simulink model "IonSatSimulation_ne_marche_pas_version_robin-lx-tavant.lab-lpp.local"  (R2019a)
settings: Solver=ode3  StartTime=0.0  StopTime=10000  FixedStep=.25  MaxStep=30  MinStep=.1  RelTol=1e-3
PreLoadFcn:
  | load('.\Data\SatConstants.mat')
model workspace (MAT data in the model file):
  MCOS : class17 (value not decoded)
  MCOS : class17 (value not decoded)
undefined symbols (not defined in the file): Angle, Axis, deg, DiscIntNeverNeededParam, IAU, km, m, mu_Earth, rad, s, sat, X, Y, Z
libraries: aerolibutil x29, sm_lib x19, nesl_utility x16, aerolibconvert2 x13, vrlib x10, simulink x9, dspmathops x8, sharedtransform x7, sharedutil x5, aerolibgravity2 x4, sharedTrackingLibrary x2, aerolibcelestial x2
(part 3 of 3)

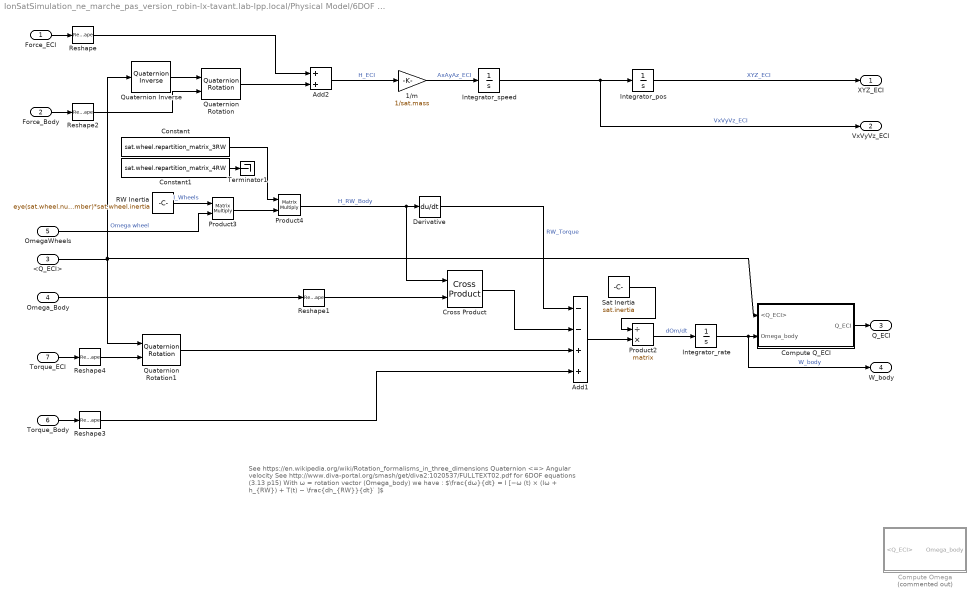
== system IonSatSimulation_ne_marche_pas_version_robin-lx-tavant.lab-lpp.local/Physical Model/6DOF in ECI frame ==
  note: See https://en.wikipedia.org/wiki/Rotation_formalisms_in_three_dimensions Quaternion <=> Angular velocity
      |
      | See http://www.diva-portal.org/smash/get/diva2:1020537/FULLTEXT02.pdf for 6DOF equations (3.13 p15)
      |
      | With ω = rotation vector (Omega_body) we have :
      |
      | $\frac{dω}{dt} = I [−ω (t) × (Iω + h_{RW}) + T(t) − \frac{dh_{RW}}{dt} ̇ ]$
  Force_ECI : Inport
  Force_Body : Inport  Port=2
  <Q_ECI> : Inport  Port=3
  "Omega_Body " : Inport  Port=4
  OmegaWheels : Inport  Port=5
  Torque_Body : Inport  Port=6
  Torque_ECI : Inport  Port=7  PortDimensions=3
  1/m : Gain  Gain=1/sat.mass
  Add1 : Sum  Inputs=--++
  Add2 : Sum
  Compute Omega : Subsystem  Commented=on
  Compute Q_ECI : Subsystem
  Constant : Constant  Value=sat.wheel.repartition_matrix_3RW
  Constant1 : Constant  Value=sat.wheel.repartition_matrix_4RW
  Cross Product : vrlib/Utilities/Cross Product
      settings: SourceProductName=Simulink
  Derivative : Derivative
  Integrator_pos : Integrator
  Integrator_rate : Integrator
  Integrator_speed : Integrator
  Product2 : Product  Inputs=/*  Multiplication=Matrix(*)
  Product3 : Product  Multiplication=Matrix(*)
  Product4 : Product  Multiplication=Matrix(*)
  Quaternion Inverse : aerolibutil/Quaternion Inverse
      settings: SourceProductName=Aerospace Blockset
  Quaternion Rotation : aerolibutil/Quaternion Rotation
  Quaternion Rotation1 : aerolibutil/Quaternion Rotation
  RW Inertia : Constant  Value=eye(sat.wheel.number)*sat.wheel.inertia
  Reshape{,1..4} (5 alike) : Reshape  OutputDimensionality=Column vector (2-D)
  Sat Inertia : Constant  Value=sat.inertia
  Terminator1 : Terminator
  XYZ_ECI : Outport
  VxVyVz_ECI : Outport  Port=2
  Q_ECI : Outport  Port=3
  W_body : Outport  Port=4
  wires:
  Product2/1 -> Integrator_rate/1  "dOm/dt"
  Product3/1 -> Product4/2
  Sat Inertia/1 -> Product2/1
  Add1/1 -> Product2/2
  Cross Product/1 -> Add1/2
  "Omega_Body "/1 -> Reshape1/1
  Integrator_rate/1 -> W_body/1, Compute Q_ECI/2(Omega_body)  "W_body"
  RW Inertia/1 -> Product3/1  "I_Wheels"
  Torque_Body/1 -> Reshape3/1
  Derivative/1 -> Add1/1  "RW_Torque"
  OmegaWheels/1 -> Product3/2  "Omega wheel"
  Compute Q_ECI/1(Q_ECI) -> Q_ECI/1
  1/m/1 -> Integrator_speed/1  "AxAyAz_ECI"
  Integrator_pos/1 -> XYZ_ECI/1  "XYZ_ECI"
  Integrator_speed/1 -> VxVyVz_ECI/1, Integrator_pos/1  "VxVyVz_ECI"
  Force_Body/1 -> Reshape2/1
  Quaternion Inverse/1 -> Quaternion Rotation/1
  Add2/1 -> 1/m/1  "H_ECI"
  Quaternion Rotation/1 -> Add2/2
  Force_ECI/1 -> Reshape/1
  Torque_ECI/1 -> Reshape4/1
  <Q_ECI>/1 -> Quaternion Rotation1/1, Quaternion Inverse/1, Compute Q_ECI/1(<Q_ECI>)
  Quaternion Rotation1/1 -> Add1/3
  Constant1/1 -> Terminator1/1
  Constant/1 -> Product4/1
  Reshape/1 -> Add2/1
  Reshape2/1 -> Quaternion Rotation/2
  Reshape3/1 -> Add1/4
  Reshape4/1 -> Quaternion Rotation1/2
  Product4/1 -> Cross Product/1, Derivative/1  "H_RW_Body"
  Reshape1/1 -> Cross Product/2

== system IonSatSimulation_ne_marche_pas_version_robin-lx-tavant.lab-lpp.local/Physical Model/Magnetorquer physics ==
  note: On pourrait aussi changer les blocs
      | magnétocoupleurs pour sortir les intensités
  Mag vector command : Inport
  B_IGRF_body (vecteur) : Inport  Port=2
  Add1 : Sum  Inputs=+++
  Cross Product : vrlib/Utilities/Cross Product
      settings: SourceProductName=Simulink
  Demux : Demux  Outputs=3
  Magnétocoupleur 1 : Subsystem
  Magnétocoupleur 2 : Subsystem
  Magnétocoupleur 3 : Subsystem
  Couple (vect) : Outport  PortDimensions=3
  Real mag moments vector : Outport  Port=2
  wires:
  Add1/1 -> Real mag moments vector/1, Cross Product/1  "M_real"
  Demux/1 -> Magnétocoupleur 1/1(m_in (scalar))
  Demux/2 -> Magnétocoupleur 2/1(m_in (scalar))
  Demux/3 -> Magnétocoupleur 3/1(m_in (scalar))
  Mag vector command/1 -> Demux/1
  Magnétocoupleur 2/1(m_out (vect)) -> Add1/2
  Magnétocoupleur 1/1(m_out (vect)) -> Add1/1
  Magnétocoupleur 3/1(m_out (vect)) -> Add1/3
  Cross Product/1 -> Couple (vect)/1  "T_body"
  B_IGRF_body (vecteur)/1 -> Cross Product/2

== system IonSatSimulation_ne_marche_pas_version_robin-lx-tavant.lab-lpp.local/Physical Model/RW physics ==
  RW command : Inport
  Demux : Demux  Outputs=3
  Mux : Mux  Inputs=3
  Transfer Fcn : TransferFcn  Denominator=[1 1]
  Transfer Fcn1 : TransferFcn  Denominator=[1 1]
  Transfer Fcn2 : TransferFcn  Denominator=[1 1]
  RW speed : Outport
  wires:
  Demux/3 -> Transfer Fcn2/1
  Demux/2 -> Transfer Fcn1/1
  Transfer Fcn2/1 -> Mux/3
  Transfer Fcn1/1 -> Mux/2
  Demux/1 -> Transfer Fcn/1
  Transfer Fcn/1 -> Mux/1
  RW command/1 -> Demux/1
  Mux/1 -> RW speed/1

== system IonSatSimulation_ne_marche_pas_version_robin-lx-tavant.lab-lpp.local/Physical Model/Spherical Harmonic Gravity ==
  note: Slower subsytem because it's too slow
  XYZ_ECI : Inport
  Time_UTC : Inport  Port=2
  ECI to ECEF IAU-2000/2006 : MATLAB Function  TreatAsAtomicUnit=on
  Product : Product  Multiplication=Matrix(*)
  Product1 : Product  Inputs=/*  Multiplication=Matrix(*)
  Spherical Harmonic Gravity Model : aerolibgravity2/Spherical Harmonic Gravity Model  units=Metric (MKS)  degree=100  action=Warning  ptype=EGM2008  datafile='aerogmm2b.mat'
      settings: SourceProductName=Aerospace Blockset  SourceProductBaseCode=AE
  Transpose : Math  Operator=transpose  SaturateOnIntegerOverflow=on
  g_ECI (m/s²) : Outport  VectorParamsAs1DForOutWhenUnconnected=on
  wires:
  ECI to ECEF IAU-2000/2006/1(DCM) -> Product1/1, Product/1
  Transpose/1 -> Product1/2
  Product/1 -> Spherical Harmonic Gravity Model/1
  Spherical Harmonic Gravity Model/1 -> Transpose/1
  XYZ_ECI/1 -> Product/2
  Product1/1 -> g_ECI (m/s²)/1
  Time_UTC/1 -> ECI to ECEF IAU-2000/2006/1(Time_UTC)

== system IonSatSimulation_ne_marche_pas_version_robin-lx-tavant.lab-lpp.local/Physical Model/Thruster ==
  On/Off (Boolean) : Inport  OutDataTypeStr=boolean
  Constant : Constant  Value=0
  Cross Product : vrlib/Utilities/Cross Product
      settings: SourceProductName=Simulink
  If : If  IfExpression=u1
  If Action Subsystem : Subsystem  TreatAsAtomicUnit=on
  If Action Subsystem1 : Subsystem  TreatAsAtomicUnit=on
  Merge : Merge
  Product : Product
  Thruster Force : Constant  Value=sat.thruster.force
  unit vector of thrust : Constant  Value=sat.thruster.dir
  vector G-Thrust point : Constant  Value=sat.thruster.point
  Force (G_sat) : Outport
  Moment (G_sat) : Outport  Port=2
  wires:
  Product/1 -> Force (G_sat)/1, Cross Product/2
  vector G-Thrust point/1 -> Cross Product/1
  unit vector of thrust/1 -> Product/1
  Cross Product/1 -> Moment (G_sat)/1
  Thruster Force/1 -> If Action Subsystem/1(In1)
  On/Off (Boolean)/1 -> If/1
  If/1 -> If Action Subsystem/Action
  If/2 -> If Action Subsystem1/Action
  If Action Subsystem1/1(Out1) -> Merge/2
  If Action Subsystem/1(Out1) -> Merge/1
  Merge/1 -> Product/2
  Constant/1 -> If Action Subsystem1/1(In1)

== system IonSatSimulation_ne_marche_pas_version_robin-lx-tavant.lab-lpp.local/Sensors/MEMS Gyro ==
  note: Voir ICD sur le CubeControl (pas 100% sur néanmoins)
  U : Inport
  Bus Selector4 : BusSelector  OutputSignals=W_body
  Constant : Constant  Value=[sat.sensors.gyro_bias sat.sensors.gyro_bias sat.sensors.gyro_bias]
  Random Number : RandomNumber  Mean=[0 0 0]  Variance=sat.sensors.mag_sigma*sat.sensors.mag_sigma  Seed=[0 5 355]  SampleTime=1
  Reshape : Reshape  OutputDimensionality=Column vector (2-D)
  Reshape1 : Reshape  OutputDimensionality=Column vector (2-D)
  Sum : Sum  Inputs=|++
  Sum1 : Sum  Inputs=|++
  W_Body_meas : Outport
  wires:
  U/1 -> Bus Selector4/1
  Random Number/1 -> Reshape/1
  Sum/1 -> Sum1/1
  Reshape/1 -> Sum/2  "Noise"
  Bus Selector4/1 -> Sum/1  "<W_body>"
  Sum1/1 -> W_Body_meas/1
  Constant/1 -> Reshape1/1
  Reshape1/1 -> Sum1/2  "Bias"

== system IonSatSimulation_ne_marche_pas_version_robin-lx-tavant.lab-lpp.local/Sensors/Magnetometer ==
  note: Valeur constructeur : 1-sigma = 50nT
  U : Inport
  B_IGRF_ECI : Inport  Port=2
  Bus Selector : BusSelector  OutputSignals=Q_ECI
  Quaternion Rotation : aerolibutil/Quaternion Rotation
  Random Number : RandomNumber  Mean=[0 0 0]  Variance=sat.sensors.mag_sigma*sat.sensors.mag_sigma  Seed=[0 5 355]  SampleTime=1
  Reshape : Reshape  OutputDimensionality=Column vector (2-D)
  Sum : Sum  Inputs=|++
  B_Body_meas : Outport
  wires:
  B_IGRF_ECI/1 -> Quaternion Rotation/2
  Random Number/1 -> Reshape/1
  Quaternion Rotation/1 -> Sum/1  "B_IGRF_body"
  Sum/1 -> B_Body_meas/1
  Reshape/1 -> Sum/2
  U/1 -> Bus Selector/1
  Bus Selector/1 -> Quaternion Rotation/1  "<Q_ECI>"

== system IonSatSimulation_ne_marche_pas_version_robin-lx-tavant.lab-lpp.local/Sensors/Sun Sensor (Coarse) ==
  note: Tests if we are not in eclipse
  note: Test d'eclipse (true = soleil visible)
  note: Two sensors because the top-camera has a 3-sigma=0.2° wheread the coarse sun sensors have sigma = 10°
  Sat-Sun_ECI : Inport
  U : Inport  Port=2
  Bus Selector : BusSelector  OutputSignals=Q_ECI,XYZ_ECI
  Constant : Constant  Value=true
  Constant1 : Constant  Value=false
  Dot Product : DotProduct  InputSameDT=on  OutDataTypeStr=Inherit: Inherit via internal rule
  Quaternion Rotation : aerolibutil/Quaternion Rotation
  Quaternion Rotation1 : aerolibutil/Quaternion Rotation
  Random Number : RandomNumber  Mean=[0 0 0]  Variance=sat.sensors.sun_coarse_sigma*sat.sensors.sun_coarse_sigma  Seed=[0 5 355]  SampleTime=1  VectorParams1D=off
  Rotation Angles to Quaternions : sharedtransform/Rotation Angles to Quaternions  rotationOrder=ZYX  aMode=aMode
      settings: SourceProductName=Aerospace Blockset  SourceProductBaseCode=AE
  Switch1 : Switch  Criteria=u2 > Threshold
  Sat-Sun_coarse_body_meas : Outport
  Sensor active (bool) : Outport  Port=2
  wires:
  Rotation Angles to Quaternions/1 -> Quaternion Rotation/1
  Quaternion Rotation/1 -> Sat-Sun_coarse_body_meas/1
  U/1 -> Bus Selector/1
  Sat-Sun_ECI/1 -> Dot Product/1, Quaternion Rotation1/2
  Bus Selector/1 -> Quaternion Rotation1/1  "<Q_ECI>"
  Quaternion Rotation1/1 -> Quaternion Rotation/2  "Sat_Sun_body"
  Bus Selector/2 -> Dot Product/2  "<XYZ_ECI>"
  Dot Product/1 -> Switch1/2
  Constant/1 -> Switch1/1
  Constant1/1 -> Switch1/3
  Switch1/1 -> Sensor active (bool)/1
  Random Number/1 -> Rotation Angles to Quaternions/1

== system IonSatSimulation_ne_marche_pas_version_robin-lx-tavant.lab-lpp.local/Sensors/Sun Sensor (Sun sensor) ==
  note: Tests if the camera is seeing the sun
  note: Test d'eclipse
  note: Two sensors because the top-camera has a 3-sigma=0.2° wheread the coarse sun sensors have sigma = 10°
  note: Valeur constructeur : 3-sigma = 0.2°
      | Donc sigma = 0.066° = 0.001164 rad
  Sat-Sun_ECI : Inport
  U : Inport  Port=2
  AND : Logic  IconShape=distinctive  AllPortsSameDT=off  OutDataTypeStr=boolean
  Bus Selector : BusSelector  OutputSignals=Q_ECI,XYZ_ECI
  Constant : Constant  Value=true
  Constant1 : Constant  Value=false
  Constant3 : Constant  Value=true
  Constant4 : Constant  Value=false
  Demux : Demux  Outputs=3
  Dot Product : DotProduct  InputSameDT=on  OutDataTypeStr=Inherit: Inherit via internal rule
  Quaternion Rotation : aerolibutil/Quaternion Rotation
  Quaternion Rotation1 : aerolibutil/Quaternion Rotation
  Random Number : RandomNumber  Mean=[0 0 0]  Variance=sat.sensors.sun_sigma*sat.sensors.sun_sigma  Seed=[0 5 355]  SampleTime=1  VectorParams1D=off
  Rotation Angles to Quaternions : sharedtransform/Rotation Angles to Quaternions  rotationOrder=ZYX  aMode=aMode
      settings: SourceProductName=Aerospace Blockset  SourceProductBaseCode=AE
  Switch : Switch  Criteria=u2 > Threshold
  Switch1 : Switch  Criteria=u2 > Threshold
  Terminator : Terminator
  Terminator1 : Terminator
  Sat-Sun_precise_body_meas : Outport
  Sensor active (bool) : Outport  Port=2
  wires:
  Switch/1 -> AND/1
  Rotation Angles to Quaternions/1 -> Quaternion Rotation/1
  Quaternion Rotation/1 -> Sat-Sun_precise_body_meas/1
  U/1 -> Bus Selector/1
  Sat-Sun_ECI/1 -> Dot Product/1, Quaternion Rotation1/2
  Bus Selector/1 -> Quaternion Rotation1/1  "<Q_ECI>"
  Quaternion Rotation1/1 -> Demux/1, Quaternion Rotation/2  "Sat_Sun_body"
  Demux/3 -> Switch/2
  Constant3/1 -> Switch/1
  Demux/2 -> Terminator/1
  Demux/1 -> Terminator1/1
  Bus Selector/2 -> Dot Product/2  "<XYZ_ECI>"
  Dot Product/1 -> Switch1/2
  Constant/1 -> Switch1/1
  Constant1/1 -> Switch1/3
  Switch1/1 -> AND/2
  AND/1 -> Sensor active (bool)/1
  Random Number/1 -> Rotation Angles to Quaternions/1
  Constant4/1 -> Switch/3

== system IonSatSimulation_ne_marche_pas_version_robin-lx-tavant.lab-lpp.local/Controller/B-dot choice1/Switch Case Action Subsystem3 ==
  In1 : Inport
  Action Port : ActionPort  ActionPortLabel=if(u1 > 0)
  Out1 : Outport
  wires:
  In1/1 -> Out1/1

== system IonSatSimulation_ne_marche_pas_version_robin-lx-tavant.lab-lpp.local/Controller/B-dot choice1/Switch Case Action Subsystem4 ==
  In1 : Inport
  Action Port : ActionPort  ActionPortLabel=else
  Out1 : Outport
  wires:
  In1/1 -> Out1/1

== system IonSatSimulation_ne_marche_pas_version_robin-lx-tavant.lab-lpp.local/Controller/B-dot choice2/Switch Case Action Subsystem3 ==
  In1 : Inport
  Action Port : ActionPort  ActionPortLabel=if(u1 > 0)
  Out1 : Outport
  wires:
  In1/1 -> Out1/1

== system IonSatSimulation_ne_marche_pas_version_robin-lx-tavant.lab-lpp.local/Controller/B-dot choice2/Switch Case Action Subsystem4 ==
  In1 : Inport
  Action Port : ActionPort  ActionPortLabel=else
  Out1 : Outport
  wires:
  In1/1 -> Out1/1

== system IonSatSimulation_ne_marche_pas_version_robin-lx-tavant.lab-lpp.local/Controller/PID (nominal command)/Command Magnetic moments computation ==
  note: Moment magnétique de commande M :
      |
      | $M_c = \frac{1}{B²}\vec{B} \wedge\vec{T_P}$
      |
      | Avec Tp couple projeté dans le plan orthogonal à B
      | $T_P=\vec{T}-\frac{1}{B²}(\vec{T}\cdot\vec{B})\vec{B}$
  Command (vect) : Inport  OutDataTypeStr=double
  B_IGRF_body (vect) : Inport  Port=2  OutDataTypeStr=double
  h1 (vect) : Inport  Port=3
  h2 (vect) : Inport  Port=4
  h3 (vect) : Inport  Port=5
  Cross Product : vrlib/Utilities/Cross Product
      settings: SourceProductName=Simulink
  Dot Product : DotProduct  InputSameDT=on  OutDataTypeStr=Inherit: Inherit via internal rule
  Global magnetic moment computation : Subsystem
  Mux : Mux  Inputs=3
  Product1 : Product  Inputs=*/
  Reshape : Reshape  OutputDimensionality=Column vector (2-D)
  Reshape1 : Reshape  OutputDimensionality=Column vector (2-D)
  Mag vector command : Outport
  wires:
  B_IGRF_body (vect)/1 -> Reshape1/1  "B_Body"
  Command (vect)/1 -> Reshape/1  "T_Body"
  h1 (vect)/1 -> Global magnetic moment computation/2(In2)
  h2 (vect)/1 -> Global magnetic moment computation/3(In3)
  h3 (vect)/1 -> Global magnetic moment computation/4(In4)
  Global magnetic moment computation/2(magnetic moment 2 (scalar)) -> Mux/2  "magnetic moment 2"
  Global magnetic moment computation/3(magnetic moment 3 (scalar)) -> Mux/3  "magnetic moment 3"
  Global magnetic moment computation/1(magnetic moment 1 (scalar)) -> Mux/1  "magnetic moment 1"
  Mux/1 -> Mag vector command/1
  Reshape1/1 -> Cross Product/1, Dot Product/2, Dot Product/1
  Cross Product/1 -> Product1/1
  Product1/1 -> Global magnetic moment computation/1(In1)  "Mc"
  Dot Product/1 -> Product1/2  "B^2"
  Reshape/1 -> Cross Product/2  "Tp"

== system IonSatSimulation_ne_marche_pas_version_robin-lx-tavant.lab-lpp.local/Controller/PID (nominal command)/Extract Vect ==
  Qr : Inport
  Demux : Demux
  Mux1 : Mux  Inputs=3
  Product : Product
  Reshape : Reshape  OutputDimensionality=Column vector (2-D)
  Sign : Signum
  Qvect : Outport
  wires:
  Demux/2 -> Mux1/1
  Demux/4 -> Mux1/3
  Demux/3 -> Mux1/2
  Demux/1 -> Sign/1
  Qr/1 -> Demux/1
  Mux1/1 -> Product/2
  Product/1 -> Reshape/1
  Sign/1 -> Product/1
  Reshape/1 -> Qvect/1

== system IonSatSimulation_ne_marche_pas_version_robin-lx-tavant.lab-lpp.local/Controller/PID (nominal command)/RW1 ==
  note: Entrées:
      | - Moment de commande (déjà projeté sur l'axe de la roue...)
      | Sorties:
      | - Omega de commande à appliquer
  Mc (scalar) : Inport
  Discrete-Time Integrator : DiscreteIntegrator  IntegratorMethod=Integration: Trapezoidal  SampleTime=-1  ICPrevOutput=DiscIntNeverNeededParam  ICPrevScaledInput=DiscIntNeverNeededParam
  Divide : Product  Inputs=*/
  Saturation_speed : Saturate  UpperLimit=sat.wheel.max_speed  LowerLimit=- sat.wheel.max_speed
  Torque_sat : Saturate  UpperLimit=sat.wheel.max_torque  LowerLimit=- sat.wheel.max_torque
  Wheel Inertia : Constant  Value=sat.wheel.max_sigma/sat.wheel.max_speed
  Omega_C (scalar) : Outport  VectorParamsAs1DForOutWhenUnconnected=on
  wires:
  Wheel Inertia/1 -> Divide/2
  Divide/1 -> Discrete-Time Integrator/1  "dw/dt"
  Discrete-Time Integrator/1 -> Saturation_speed/1
  Torque_sat/1 -> Divide/1  "Torque (scal)"
  Saturation_speed/1 -> Omega_C (scalar)/1
  Mc (scalar)/1 -> Torque_sat/1

== system IonSatSimulation_ne_marche_pas_version_robin-lx-tavant.lab-lpp.local/Controller/PID (nominal command)/RW2 ==
  note: Entrées:
      | - Moment de commande (déjà projeté sur l'axe de la roue...)
      | Sorties:
      | - Omega de commande à appliquer
  Mc (scalar) : Inport
  Discrete-Time Integrator : DiscreteIntegrator  IntegratorMethod=Integration: Trapezoidal  SampleTime=-1  ICPrevOutput=DiscIntNeverNeededParam  ICPrevScaledInput=DiscIntNeverNeededParam
  Divide : Product  Inputs=*/
  Saturation_speed : Saturate  UpperLimit=sat.wheel.max_speed  LowerLimit=- sat.wheel.max_speed
  Torque_sat : Saturate  UpperLimit=sat.wheel.max_torque  LowerLimit=- sat.wheel.max_torque
  Wheel Inertia : Constant  Value=sat.wheel.max_sigma/sat.wheel.max_speed
  Omega_C (scalar) : Outport  VectorParamsAs1DForOutWhenUnconnected=on
  wires:
  Wheel Inertia/1 -> Divide/2
  Divide/1 -> Discrete-Time Integrator/1  "dw/dt"
  Discrete-Time Integrator/1 -> Saturation_speed/1
  Torque_sat/1 -> Divide/1  "Torque (scal)"
  Saturation_speed/1 -> Omega_C (scalar)/1
  Mc (scalar)/1 -> Torque_sat/1

== system IonSatSimulation_ne_marche_pas_version_robin-lx-tavant.lab-lpp.local/Controller/PID (nominal command)/RW3 ==
  note: Entrées:
      | - Moment de commande (déjà projeté sur l'axe de la roue...)
      | Sorties:
      | - Omega de commande à appliquer
  Mc (scalar) : Inport
  Discrete-Time Integrator : DiscreteIntegrator  IntegratorMethod=Integration: Trapezoidal  SampleTime=-1  ICPrevOutput=DiscIntNeverNeededParam  ICPrevScaledInput=DiscIntNeverNeededParam
  Divide : Product  Inputs=*/
  Saturation_speed : Saturate  UpperLimit=sat.wheel.max_speed  LowerLimit=- sat.wheel.max_speed
  Torque_sat : Saturate  UpperLimit=sat.wheel.max_torque  LowerLimit=- sat.wheel.max_torque
  Wheel Inertia : Constant  Value=sat.wheel.max_sigma/sat.wheel.max_speed
  Omega_C (scalar) : Outport  VectorParamsAs1DForOutWhenUnconnected=on
  wires:
  Wheel Inertia/1 -> Divide/2
  Divide/1 -> Discrete-Time Integrator/1  "dw/dt"
  Discrete-Time Integrator/1 -> Saturation_speed/1
  Torque_sat/1 -> Divide/1  "Torque (scal)"
  Saturation_speed/1 -> Omega_C (scalar)/1
  Mc (scalar)/1 -> Torque_sat/1

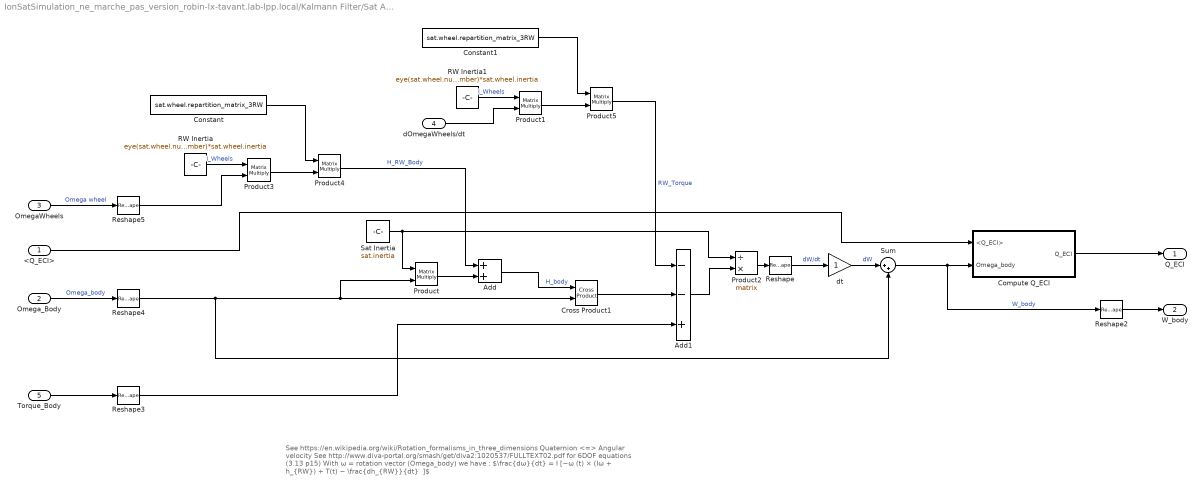
== system IonSatSimulation_ne_marche_pas_version_robin-lx-tavant.lab-lpp.local/Kalmann Filter/Sat Attitude/6DOF in ECI frame ==
  note: See https://en.wikipedia.org/wiki/Rotation_formalisms_in_three_dimensions Quaternion <=> Angular velocity
      |
      | See http://www.diva-portal.org/smash/get/diva2:1020537/FULLTEXT02.pdf for 6DOF equations (3.13 p15)
      |
      | With ω = rotation vector (Omega_body) we have :
      |
      | $\frac{dω}{dt} = I [−ω (t) × (Iω + h_{RW}) + T(t) − \frac{dh_{RW}}{dt} ̇ ]$
  <Q_ECI> : Inport
  "Omega_Body " : Inport  Port=2
  OmegaWheels : Inport  Port=3
  dOmegaWheels/dt : Inport  Port=4
  Torque_Body : Inport  Port=5
  Add : Sum
  Add1 : Sum  Inputs=--+
  Compute Q_ECI : Subsystem
  Constant : Constant  Value=sat.wheel.repartition_matrix_3RW
  Constant1 : Constant  Value=sat.wheel.repartition_matrix_3RW
  Cross Product1 : vrlib/Utilities/Cross Product
      settings: SourceProductName=Simulink
  Product{,1,3..5} (5 alike) : Product  Multiplication=Matrix(*)
  Product2 : Product  Inputs=/*  Multiplication=Matrix(*)
  RW Inertia : Constant  Value=eye(sat.wheel.number)*sat.wheel.inertia
  RW Inertia1 : Constant  Value=eye(sat.wheel.number)*sat.wheel.inertia
  Reshape : Reshape
  Reshape2 : Reshape
  Reshape3 : Reshape  OutputDimensionality=Column vector (2-D)
  Reshape4 : Reshape  OutputDimensionality=Column vector (2-D)
  Reshape5 : Reshape  OutputDimensionality=Column vector (2-D)
  Sat Inertia : Constant  Value=sat.inertia
  Sum : Sum  Inputs=|++
  dt : Gain
  Q_ECI : Outport
  W_body : Outport  Port=2
  wires:
  Product2/1 -> Reshape/1
  Product3/1 -> Product4/2
  Sat Inertia/1 -> Product/1, Product2/1
  Add/1 -> Cross Product1/1  "H_body"
  Add1/1 -> Product2/2
  Cross Product1/1 -> Add1/2
  "Omega_Body "/1 -> Reshape4/1  "Omega_body"
  Product/1 -> Add/2
  RW Inertia/1 -> Product3/1  "I_Wheels"
  Torque_Body/1 -> Reshape3/1
  Product5/1 -> Add1/1  "RW_Torque"
  OmegaWheels/1 -> Reshape5/1  "Omega wheel"
  Constant/1 -> Product4/1
  Product4/1 -> Add/1  "H_RW_Body"
  Reshape3/1 -> Add1/3
  Reshape/1 -> dt/1  "dW/dt"
  Sum/1 -> Compute Q_ECI/2(Omega_body), Reshape2/1  "W_body"
  Compute Q_ECI/1(Q_ECI) -> Q_ECI/1
  Reshape2/1 -> W_body/1
  Reshape4/1 -> Sum/2, Cross Product1/2, Product/2
  Reshape5/1 -> Product3/2
  <Q_ECI>/1 -> Compute Q_ECI/1(<Q_ECI>)
  dt/1 -> Sum/1  "dW"
  dOmegaWheels/dt/1 -> Product1/2
  Constant1/1 -> Product5/1
  Product1/1 -> Product5/2
  RW Inertia1/1 -> Product1/1  "I_Wheels"

== system IonSatSimulation_ne_marche_pas_version_robin-lx-tavant.lab-lpp.local/Kalmann Filter/Sat Attitude/Magnetorquer physics ==
  note: On pourrait aussi changer les blocs
      | magnétocoupleurs pour sortir les intensités
  Mag vector command : Inport
  B_IGRF_body (vecteur) : Inport  Port=2
  Add1 : Sum  Inputs=+++
  Cross Product : vrlib/Utilities/Cross Product
      settings: SourceProductName=Simulink
  Demux : Demux  Outputs=3
  Magnétocoupleur 1 : Subsystem
  Magnétocoupleur 2 : Subsystem
  Magnétocoupleur 3 : Subsystem
  Couple (vect) : Outport
  wires:
  Add1/1 -> Cross Product/1  "M_real"
  Demux/1 -> Magnétocoupleur 1/1(m_in (scalar))
  Demux/2 -> Magnétocoupleur 2/1(m_in (scalar))
  Demux/3 -> Magnétocoupleur 3/1(m_in (scalar))
  Mag vector command/1 -> Demux/1
  Magnétocoupleur 2/1(m_out (vect)) -> Add1/2
  Magnétocoupleur 1/1(m_out (vect)) -> Add1/1
  Magnétocoupleur 3/1(m_out (vect)) -> Add1/3
  Cross Product/1 -> Couple (vect)/1  "T_body"
  B_IGRF_body (vecteur)/1 -> Cross Product/2

== system IonSatSimulation_ne_marche_pas_version_robin-lx-tavant.lab-lpp.local/Kalmann Filter/Sat Attitude1/Compute Q_ECI ==
  note: https://arxiv.org/pdf/0811.2889.pdf
      | $ω = 2q^*\frac{dq}{dt}$ (13)
      |
      | $\frac{dq}{dt} = \frac{1}{2} q * ω$ (14)
  <Q_ECI> : Inport
  Omega_body : Inport  Port=2
  Gain : Gain  Gain=1/2
  Ground : Ground
  Mux : Mux  Inputs=2
  Quaternion Multiplication : aerolibutil/Quaternion Multiplication
  Quaternion Normalize : sharedutil/Quaternion Normalize  aMode=aMode
      settings: SourceProductName=Aerospace Blockset  SourceProductBaseCode=AE
  Sum : Sum  Inputs=|++
  dt : Gain
  Q_ECI : Outport
  wires:
  Quaternion Multiplication/1 -> Gain/1
  Omega_body/1 -> Mux/2
  Ground/1 -> Mux/1
  Mux/1 -> Quaternion Multiplication/2
  Quaternion Normalize/1 -> Q_ECI/1  "Q_ECI"
  Sum/1 -> Quaternion Normalize/1
  <Q_ECI>/1 -> Quaternion Multiplication/1, Sum/1
  Gain/1 -> dt/1  "dQ"
  dt/1 -> Sum/2

== system IonSatSimulation_ne_marche_pas_version_robin-lx-tavant.lab-lpp.local/Physical Model/6DOF in ECI frame/Compute Omega ==
  note: https://arxiv.org/pdf/0811.2889.pdf
      | $ω = 2q^*\frac{dq}{dt}$ (13)
  <Q_ECI> : Inport
  Demux : Demux  Outputs=2
  Derivative : Derivative
  Gain : Gain  Gain=2
  Quaternion Conjugate : aerolibutil/Quaternion Conjugate
      settings: SourceProductName=Aerospace Blockset  SourceProductBaseCode=AE
  Quaternion Multiplication : aerolibutil/Quaternion Multiplication
  Reshape : Reshape  OutputDimensionality=Column vector (2-D)
  Terminator : Terminator
  Omega_body : Outport  PortDimensions=[3 1]
  wires:
  Quaternion Multiplication/1 -> Demux/1
  <Q_ECI>/1 -> Derivative/1, Quaternion Conjugate/1
  Demux/1 -> Terminator/1
  Demux/2 -> Reshape/1
  Reshape/1 -> Gain/1
  Gain/1 -> Omega_body/1
  Quaternion Conjugate/1 -> Quaternion Multiplication/1
  Derivative/1 -> Quaternion Multiplication/2

== system IonSatSimulation_ne_marche_pas_version_robin-lx-tavant.lab-lpp.local/Physical Model/6DOF in ECI frame/Compute Q_ECI ==
  note: https://arxiv.org/pdf/0811.2889.pdf
      | $ω = 2q^*\frac{dq}{dt}$ (13)
      |
      | $\frac{dq}{dt} = \frac{1}{2} q * ω$ (14)
  <Q_ECI> : Inport
  Omega_body : Inport  Port=2
  Gain : Gain  Gain=1/2
  Ground : Ground
  Integrator_quat : Integrator  InitialCondition=[1 0 0 0]
  Mux : Mux  Inputs=2
  Quaternion Multiplication : aerolibutil/Quaternion Multiplication
  Quaternion Normalize : sharedutil/Quaternion Normalize  aMode=aMode
      settings: SourceProductName=Aerospace Blockset  SourceProductBaseCode=AE
  Q_ECI : Outport
  wires:
  Quaternion Multiplication/1 -> Gain/1
  Omega_body/1 -> Mux/2
  Ground/1 -> Mux/1
  Mux/1 -> Quaternion Multiplication/2
  <Q_ECI>/1 -> Quaternion Multiplication/1
  Integrator_quat/1 -> Quaternion Normalize/1
  Gain/1 -> Integrator_quat/1
  Quaternion Normalize/1 -> Q_ECI/1  "Q_ECI"

== system IonSatSimulation_ne_marche_pas_version_robin-lx-tavant.lab-lpp.local/Physical Model/Magnetorquer physics/Magnétocoupleur 1 ==
  note: les grounds représentant les limites en
      |  moment magnétique du magnétocoupleur (lié à l'intensité)
      | A définir
  m_in (scalar) : Inport
  Constant1 : Constant  Value=sat.mag_t.max_mm1
  Constant2 : Constant  Value=- sat.mag_t.max_mm1
  Constant6 : Constant  Value=sat.mag_t.axe1
  Product : Product
  Saturation Dynamic : simulink/Discontinuities/Saturation Dynamic  OutMin=[]  OutMax=[]  OutDataTypeStr=Inherit: Same as second input  OutDataType=fixdt(1, 16)  OutScaling=2^-10  DoSatur=off
  m_out (vect) : Outport
  wires:
  m_in (scalar)/1 -> Saturation Dynamic/2
  Constant2/1 -> Saturation Dynamic/3
  Constant1/1 -> Saturation Dynamic/1
  Saturation Dynamic/1 -> Product/1
  Product/1 -> m_out (vect)/1
  Constant6/1 -> Product/2

== system IonSatSimulation_ne_marche_pas_version_robin-lx-tavant.lab-lpp.local/Physical Model/Magnetorquer physics/Magnétocoupleur 2 ==
  note: les grounds représentant les limites en
      |  moment magnétique du magnétocoupleur (lié à l'intensité)
      | A définir
  m_in (scalar) : Inport
  Constant : Constant  Value=- sat.mag_t.max_mm2
  Constant1 : Constant  Value=sat.mag_t.max_mm2
  Constant6 : Constant  Value=sat.mag_t.axe2
  Product : Product
  Saturation Dynamic : simulink/Discontinuities/Saturation Dynamic  OutMin=[]  OutMax=[]  OutDataTypeStr=Inherit: Same as second input  OutDataType=fixdt(1, 16)  OutScaling=2^-10  DoSatur=off
  m_out (vect) : Outport
  wires:
  m_in (scalar)/1 -> Saturation Dynamic/2
  Constant/1 -> Saturation Dynamic/3
  Constant1/1 -> Saturation Dynamic/1
  Product/1 -> m_out (vect)/1
  Constant6/1 -> Product/2
  Saturation Dynamic/1 -> Product/1

== system IonSatSimulation_ne_marche_pas_version_robin-lx-tavant.lab-lpp.local/Physical Model/Magnetorquer physics/Magnétocoupleur 3 ==
  note: les grounds représentant les limites en
      |  moment magnétique du magnétocoupleur (lié à l'intensité)
      | A définir
  m_in (scalar) : Inport
  Constant1 : Constant  Value=sat.mag_t.max_mm3
  Constant2 : Constant  Value=- sat.mag_t.max_mm3
  Constant6 : Constant  Value=sat.mag_t.axe3
  Product : Product
  Saturation Dynamic : simulink/Discontinuities/Saturation Dynamic  OutMin=[]  OutMax=[]  OutDataTypeStr=Inherit: Same as second input  OutDataType=fixdt(1, 16)  OutScaling=2^-10  DoSatur=off
  m_out (vect) : Outport
  wires:
  m_in (scalar)/1 -> Saturation Dynamic/2
  Constant2/1 -> Saturation Dynamic/3
  Constant1/1 -> Saturation Dynamic/1
  Product/1 -> m_out (vect)/1
  Constant6/1 -> Product/2
  Saturation Dynamic/1 -> Product/1

== system IonSatSimulation_ne_marche_pas_version_robin-lx-tavant.lab-lpp.local/Physical Model/Thruster/If Action Subsystem ==
  In1 : Inport
  Action Port : ActionPort  ActionPortLabel=if(u1)
  Out1 : Outport  VectorParamsAs1DForOutWhenUnconnected=on
  wires:
  In1/1 -> Out1/1

== system IonSatSimulation_ne_marche_pas_version_robin-lx-tavant.lab-lpp.local/Physical Model/Thruster/If Action Subsystem1 ==
  In1 : Inport
  Action Port : ActionPort  ActionPortLabel=else
  Out1 : Outport  VectorParamsAs1DForOutWhenUnconnected=on
  wires:
  In1/1 -> Out1/1

== system IonSatSimulation_ne_marche_pas_version_robin-lx-tavant.lab-lpp.local/Controller/PID (nominal command)/Command Magnetic moments computation/Global magnetic moment computation ==
  In1 : Inport  OutDataTypeStr=double
  In2 : Inport  Port=2
  In3 : Inport  Port=3
  In4 : Inport  Port=4
  Dot Product : DotProduct  InputSameDT=on  OutDataTypeStr=Inherit: Inherit via internal rule
  Dot Product1 : DotProduct  InputSameDT=on  OutDataTypeStr=Inherit: Inherit via internal rule
  Dot Product2 : DotProduct  InputSameDT=on  OutDataTypeStr=Inherit: Inherit via internal rule
  magnetic moment 1 (scalar) : Outport  VectorParamsAs1DForOutWhenUnconnected=on
  magnetic moment 2 (scalar) : Outport  Port=2  VectorParamsAs1DForOutWhenUnconnected=on
  magnetic moment 3 (scalar) : Outport  Port=3  VectorParamsAs1DForOutWhenUnconnected=on
  wires:
  In1/1 -> Dot Product2/1, Dot Product1/1, Dot Product/1
  In2/1 -> Dot Product/2
  In3/1 -> Dot Product1/2
  In4/1 -> Dot Product2/2
  Dot Product/1 -> magnetic moment 1 (scalar)/1
  Dot Product1/1 -> magnetic moment 2 (scalar)/1
  Dot Product2/1 -> magnetic moment 3 (scalar)/1

== system IonSatSimulation_ne_marche_pas_version_robin-lx-tavant.lab-lpp.local/Kalmann Filter/Sat Attitude/6DOF in ECI frame/Compute Q_ECI ==
  note: https://arxiv.org/pdf/0811.2889.pdf
      | $ω = 2q^*\frac{dq}{dt}$ (13)
      |
      | $\frac{dq}{dt} = \frac{1}{2} q * ω$ (14)
  <Q_ECI> : Inport
  Omega_body : Inport  Port=2
  Gain : Gain  Gain=1/2
  Ground : Ground
  Mux : Mux  Inputs=2
  Quaternion Multiplication : aerolibutil/Quaternion Multiplication
  Quaternion Normalize : sharedutil/Quaternion Normalize  aMode=aMode
      settings: SourceProductName=Aerospace Blockset  SourceProductBaseCode=AE
  Sum : Sum  Inputs=|++
  dt : Gain
  Q_ECI : Outport
  wires:
  Quaternion Multiplication/1 -> Gain/1
  Omega_body/1 -> Mux/2
  Ground/1 -> Mux/1
  Mux/1 -> Quaternion Multiplication/2
  Quaternion Normalize/1 -> Q_ECI/1  "Q_ECI"
  Sum/1 -> Quaternion Normalize/1
  <Q_ECI>/1 -> Quaternion Multiplication/1, Sum/1
  Gain/1 -> dt/1  "dQ"
  dt/1 -> Sum/2

== system IonSatSimulation_ne_marche_pas_version_robin-lx-tavant.lab-lpp.local/Kalmann Filter/Sat Attitude/Magnetorquer physics/Magnétocoupleur 1 ==
  note: les grounds représentant les limites en
      |  moment magnétique du magnétocoupleur (lié à l'intensité)
      | A définir
  m_in (scalar) : Inport
  Constant1 : Constant  Value=sat.mag_t.max_mm1
  Constant2 : Constant  Value=- sat.mag_t.max_mm1
  Constant6 : Constant  Value=sat.mag_t.axe1
  Product : Product
  Saturation Dynamic : simulink/Discontinuities/Saturation Dynamic  OutMin=[]  OutMax=[]  OutDataTypeStr=Inherit: Same as second input  OutDataType=fixdt(1, 16)  OutScaling=2^-10  DoSatur=off
  m_out (vect) : Outport
  wires:
  m_in (scalar)/1 -> Saturation Dynamic/2
  Constant2/1 -> Saturation Dynamic/3
  Constant1/1 -> Saturation Dynamic/1
  Saturation Dynamic/1 -> Product/1
  Product/1 -> m_out (vect)/1
  Constant6/1 -> Product/2

== system IonSatSimulation_ne_marche_pas_version_robin-lx-tavant.lab-lpp.local/Kalmann Filter/Sat Attitude/Magnetorquer physics/Magnétocoupleur 2 ==
  note: les grounds représentant les limites en
      |  moment magnétique du magnétocoupleur (lié à l'intensité)
      | A définir
  m_in (scalar) : Inport
  Constant : Constant  Value=- sat.mag_t.max_mm2
  Constant1 : Constant  Value=sat.mag_t.max_mm2
  Constant6 : Constant  Value=sat.mag_t.axe2
  Product : Product
  Saturation Dynamic : simulink/Discontinuities/Saturation Dynamic  OutMin=[]  OutMax=[]  OutDataTypeStr=Inherit: Same as second input  OutDataType=fixdt(1, 16)  OutScaling=2^-10  DoSatur=off
  m_out (vect) : Outport
  wires:
  m_in (scalar)/1 -> Saturation Dynamic/2
  Constant/1 -> Saturation Dynamic/3
  Constant1/1 -> Saturation Dynamic/1
  Product/1 -> m_out (vect)/1
  Constant6/1 -> Product/2
  Saturation Dynamic/1 -> Product/1

== system IonSatSimulation_ne_marche_pas_version_robin-lx-tavant.lab-lpp.local/Kalmann Filter/Sat Attitude/Magnetorquer physics/Magnétocoupleur 3 ==
  note: les grounds représentant les limites en
      |  moment magnétique du magnétocoupleur (lié à l'intensité)
      | A définir
  m_in (scalar) : Inport
  Constant1 : Constant  Value=sat.mag_t.max_mm3
  Constant2 : Constant  Value=- sat.mag_t.max_mm3
  Constant6 : Constant  Value=sat.mag_t.axe3
  Product : Product
  Saturation Dynamic : simulink/Discontinuities/Saturation Dynamic  OutMin=[]  OutMax=[]  OutDataTypeStr=Inherit: Same as second input  OutDataType=fixdt(1, 16)  OutScaling=2^-10  DoSatur=off
  m_out (vect) : Outport
  wires:
  m_in (scalar)/1 -> Saturation Dynamic/2
  Constant2/1 -> Saturation Dynamic/3
  Constant1/1 -> Saturation Dynamic/1
  Product/1 -> m_out (vect)/1
  Constant6/1 -> Product/2
  Saturation Dynamic/1 -> Product/1

== matlab function IonSatSimulation_ne_marche_pas_version_robin-lx-tavant.lab-lpp.local/rv2orb ==
  data: r input; a output; v input; mu input; eMag output; i output; O output; o output; nu output; truLon output; argLat output; lonPer output; p output
%----------------------- Begin Code Sequence -----------------------------%
% Purpose:                                                                %
% Convert a given set of state vectors in ECI reference frame to orbital  %
% elements.                                                               %
%-------------------------------------------------------------------------%
%                                                                         %
% Inputs:                                                                 %
%--------                                                                  
%r_ECI                  [3 x N]                         Position Vector in
%                                                       ECI coordinate
%                                                       frame of reference
%
%v_ECI                  [3 x N]                         Velocity vector in
%                                                       ECI coordinate
%                                                       frame of reference
%
%mu                     double                          Gravitational Constant
%                                                       Defaults to Earth if
%                                                       not specified
% Outputs:
%---------                                                                %
%a                      [1 x N]                         Semi-Major Axis
%                                                       (km)
%
%eMag                   [1 x N]                         Eccentricity
%                                                       (unitless)
%
%i                      [1 x N]                         inclination
%                                                       (radians)
%
%O                      [1 x N]                         Right Ascention of
%                                                       the ascending node
%                                                       (radians)
%
%o                      [1 x N]                         Argument of perigee
%                                                       (radians)
%
%M                      [1 x N]                         Mean Anomaly
%                                                       (radians)
%
%truLon                 [1 x N]                         True Longitude
%                                                       (radians)
%
%argLat                 [1 x N]                         Argument of Latitude
%                                                       (radians)
%
%lonPer                 [1 x N]                         Longitude of Periapse
%                                                       (radians)
%
%p                      [1 x N]                         Semilatus Rectum
%                                                       (km)
%
% References:
%-------------
%Vallado,D. Fundamentals of Astrodynamics and Applications. 2007.
%
% Function Dependencies:
%------------------
%None
%------------------------------------------------------------------       %
% Programed by Darin Koblick  03-04-2012                                  %
% Updated to address circular equatorial orbits       12/12/2013          %
%------------------------------------------------------------------       %
function [a,eMag,i,O,o,nu,truLon,argLat,lonPer,p] = rv2orb(r,v,mu)
if ~exist('mu','var');  t = getConst(); mu = t.Earth.Mu; end
%Specific angular momentum
h = cross(r,v);
n = cross(repmat([0;0;1],[1,size(r,2)]),h); nMag = sqrt(sum(n.^2,1));
vMag = sqrt(sum(v.^2,1)); 
rMag = sqrt(sum(r.^2,1)); 
hMag = sqrt(sum(h.^2,1));
e = (1./mu).*(bsxfun(@times,(vMag.^2 - mu./rMag),r) - bsxfun(@times,dot(r,v),v)); 
eMag = sqrt(sum(e.^2,1));
zeta = (vMag.^2)./2 - mu./rMag;
%Special Procedure when we have a parabolic orbit
idx = eMag ~= 1;
a = NaN(size(eMag));
p = NaN(size(eMag));
if any(idx)
    a(idx) = -mu./(2.*zeta(idx)); 
    p = a(idx).*(1-eMag(idx).^2); 
else
    a(idx) = Inf; 
    p(idx) = (hMag(idx).^2)./mu; 
end
%Compute the angles
i = acos(h(3,:)./hMag); 
O = acos(n(1,:)./nMag);
o = acos(dot(n,e)./(nMag.*eMag));
nu = acos(dot(e,r)./(eMag.*rMag));
lonPer = acos(e(1,:)./eMag);
argLat = acos(dot(n,r)./(nMag.*rMag));
truLon = acos(r(1,:)./rMag);
%Account for those cases where satellite is in circular orbit
         O(n(1,:) == 0) = 0;
       o(dot(n,e) == 0) = 0;
    lonPer(e(1,:) == 0) = 0;
      nu(dot(e,r) == 0) = 0;
  argLat(dot(n,r) == 0) = 0;
%Apply Quadrant Checks to All Determined Angles
idx = n(2,:) < 0; if any(idx);  O(idx) = 2*pi - O(idx);  end
idx = e(3,:) < 0; if any(idx); o(idx) = 2*pi - o(idx); end
idx = dot(r,v) < 0; if any(idx); nu(idx) = 2*pi - nu(idx); end
idx = e(2,:) < 0; if any(idx); lonPer(idx) = 2*pi-lonPer(idx);  end
idx = r(3,:) < 0; if any(idx); argLat(idx) = 2*pi - argLat(idx); end
idx = r(2,:) < 0; if any(idx); truLon(idx) = 2*pi - truLon(idx); end
end

== matlab function IonSatSimulation_ne_marche_pas_version_robin-lx-tavant.lab-lpp.local/Initialize Function/orb2rv ==
  data: a input; r output; e input; i input; O input; o input; nu input; v output; truLon input; argLat input; lonPer input
%----------------------- Begin Code Sequence -----------------------------%
% Purpose:                                                                %
% Convert a given set of Keplerian Orbital Elements to state vectors in   %
% in the ECI frame of reference                                           %
%                                                                         %
%-------------------------------------------------------------------------%
%                                                                         %
% Inputs:                                                                 %
%-------- 
%a                      [1 x N]                         Semimajor axis
%                                                       (km)
%
%e                      [1 x N]                         Eccentricity Magnitude
%                                                       (unitless)
%
%i                      [1 x N]                         inclination
%                                                       (radians)
%
%O                      [1 x N]                         Right Ascention of
%                                                       the ascending node
%                                                       (radians)
%
%o                      [1 x N]                         Argument of perigee
%                                                       (radians)
%
%nu                     [1 x N]                         True Anomaly
%                                                       (radians)
%
%truLon                 [1 x N]                         True Longitude
%                                                       (radians)
%
%argLat                 [1 x N]                         Argument of Latitude
%                                                       (radians)
%
%lonPer                 [1 x N]                         Longitude of Periapse
%                                                       (radians)
%
%mu                     double                          Gravitational Constant
%                                                       Defaults to Earth if
%                                                       not specified
%
% Outputs:
%---------                                                                %
%r_ECI                  [3 x N]                         Position Vector in
%                                                       ECI coordinate
%                                                       frame of reference
%
%v_ECI                  [3 x N]                         Velocity vector in
%                                                       ECI coordinate
%                                                       frame of reference
%
% References:
%-------------
%Vallado,D. Fundamentals of Astrodynamics and Applications. 2007.
%
% Function Dependencies:
%------------------
%None
%------------------------------------------------------------------       %
% Programed by Darin Koblick  03-04-2012                                  %
%------------------------------------------------------------------       %
function [r,v] = orb2rv(a,e,i,O,o,nu,truLon,argLat,lonPer)
mu = 398600.4418;
%Make all inputs consistent w/ dimensions
a = a(:); e = e(:); i = i(:); O = O(:); o = o(:); nu = nu(:);
if e<1
    p=a*(1-e*e);
else
    p=2*a;
end
ietol = 1e-8;
idx = e < ietol & mod(i,pi) < ietol;
if any(idx); o(idx) = 0; O(idx) = 0; nu(idx) = truLon(idx); end
idx = e < ietol & mod(i,pi) > ietol;
if any(idx); o(idx) = 0; nu(idx) = argLat(idx); end
idx = e > ietol & mod(i,pi) < ietol;
if any(idx); O(idx) = 0; o(idx) = lonPer(idx); end
%Find rPQW and vPQW
rPQW = cat(2,p.*cos(nu)./(1 +e.*cos(nu)),p.*sin(nu)./(1+e.*cos(nu)),zeros(size(nu)));
vPQW = cat(2,-sqrt(mu./p).*sin(nu),sqrt(mu./p).*(e+cos(nu)),zeros(size(nu)));
%Create Transformation Matrix
PQW2IJK = NaN(3,3,size(p,1));
cO = cos(O); sO = sin(O); co = cos(o); so = sin(o); ci = cos(i); si = sin(i);
PQW2IJK(1,1,:) = cO.*co-sO.*so.*ci; PQW2IJK(1,2,:) = -cO.*so-sO.*co.*ci; PQW2IJK(1,3,:) = sO.*si;
PQW2IJK(2,1,:) = sO.*co+cO.*so.*ci; PQW2IJK(2,2,:) = -sO.*so+cO.*co.*ci; PQW2IJK(2,3,:) = -cO.*si;
PQW2IJK(3,1,:) = so.*si;            PQW2IJK(3,2,:) = co.*si;             PQW2IJK(3,3,:) = ci;
%Transform rPQW and vPQW to rECI and vECI
r = multiDimMatrixMultiply(PQW2IJK,rPQW)';  
v = multiDimMatrixMultiply(PQW2IJK,vPQW)';
end
function c = multiDimMatrixMultiply(a,b)
c = NaN(size(b));
c(:,1) = sum(bsxfun(@times,a(1,:,:),permute(b,[3 2 1])),2);
c(:,2) = sum(bsxfun(@times,a(2,:,:),permute(b,[3 2 1])),2);
c(:,3) = sum(bsxfun(@times,a(3,:,:),permute(b,[3 2 1])),2);
end

== matlab function IonSatSimulation_ne_marche_pas_version_robin-lx-tavant.lab-lpp.local/IGRF Computation block/ECI To LLA ==
  data: X_ECEF input; h output; lat output; long output
function [h, lat, long] = fcn(X_ECEF)
    h = 0;
    lat = 0;
    long = 0;
[lat, long, h] = ecef2geod(X_ECEF(1),X_ECEF(2),X_ECEF(3));

== matlab function IonSatSimulation_ne_marche_pas_version_robin-lx-tavant.lab-lpp.local/IGRF Computation block/IGRF model ==
  data: Time_UTC input; h input; magFieldVector output; lat input; long input
function magFieldVector = fcn(Time_UTC, h,lat,long)
    
magFieldVector = igrfsim(Time_UTC, h,lat,long); %output in Tesla

== matlab function IonSatSimulation_ne_marche_pas_version_robin-lx-tavant.lab-lpp.local/IGRF Computation block1/ECI To LLA ==
  data: X_ECI input; h output; Time_UTC input; lat output; long output
function [h, lat, long] = fcn(X_ECI,Time_UTC)

[h, lat, long] = eci2lla(X_ECI,Time_UTC);

== matlab function IonSatSimulation_ne_marche_pas_version_robin-lx-tavant.lab-lpp.local/IGRF Computation block1/IGRF model ==
  data: h input; magFieldVector output; lat input; long input; Time_UTC input
function magFieldVector = fcn(h,lat,long,Time_UTC)
    vect_Res=igrfmagm(h,lat,long,Time_UTC(1));
magFieldVector = vect_Res(1) * 1E-9; %output in Tesla

== matlab function IonSatSimulation_ne_marche_pas_version_robin-lx-tavant.lab-lpp.local/Time propagator/UTC to JD ==
  data: Time_UTC input; JD output
function JD = fcn(Time_UTC)

JD = Dt2jD(Time_UTC);

== matlab function IonSatSimulation_ne_marche_pas_version_robin-lx-tavant.lab-lpp.local/Time propagator/JD to UTC ==
  data: JD input; Time_UTC output
function Time_UTC = fcn(JD)
    coder.extrinsic('datetime','datevec');
    Time_UTC = [0,0,0,0,0,0];
Time_UTC =  datevec(datetime(JD,'convertfrom','juliandate'));

== matlab function IonSatSimulation_ne_marche_pas_version_robin-lx-tavant.lab-lpp.local/Physical Model/Spherical Harmonic Gravity/ECI to ECEF IAU-2000//2006 ==
  data: Time_UTC input; DCM output
function DCM = fcn(Time_UTC)
    coder.extrinsic('dcmeci2ecef');
    DCM = zeros(3,3);
DCM = dcmeci2ecef('IAU-2000/2006',Time_UTC);

== matlab function IonSatSimulation_ne_marche_pas_version_robin-lx-tavant.lab-lpp.local/IGRF Computation block/ECI to ECEF IAU-2000//2006 à remplacer par un bloc codable ==
  data: Time_UTC input; DCM output
function DCM = fcn(Time_UTC)
    coder.extrinsic('dcmeci2ecef');
    DCM = zeros(3,3);
DCM = dcmeci2ecef('IAU-2000/2006',Time_UTC);

== matlab function IonSatSimulation_ne_marche_pas_version_robin-lx-tavant.lab-lpp.local/Kalmann Filter/IGRF embedded/ECI To LLA ==
  data: X_ECEF input; h output; lat output; long output
function [h, lat, long] = fcn(X_ECEF)
    h = 0;
    lat = 0;
    long = 0;
[lat, long, h] = ecef2geod(X_ECEF(1),X_ECEF(2),X_ECEF(3));

== matlab function IonSatSimulation_ne_marche_pas_version_robin-lx-tavant.lab-lpp.local/Kalmann Filter/IGRF embedded/ECI to ECEF IAU-2000//2006 à remplacer par un bloc codable ==
  data: Time_UTC input; DCM output
function DCM = fcn(Time_UTC)
    coder.extrinsic('dcmeci2ecef');
    DCM = zeros(3,3);
DCM = dcmeci2ecef('IAU-2000/2006',Time_UTC);

== matlab function IonSatSimulation_ne_marche_pas_version_robin-lx-tavant.lab-lpp.local/Kalmann Filter/IGRF embedded/IGRF model ==
  data: Time_UTC input; h input; magFieldVector output; lat input; long input
function magFieldVector = fcn(Time_UTC, h,lat,long)
    
magFieldVector = igrfsim(Time_UTC, h,lat,long); %output in Tesla
